simulink model "RecvR4sStEnCtrl1"  (R2024b)
settings: Solver=FixedStepDiscrete  StartTime=0.0  StopTime=10.0  FixedStep=0.01  RelTol=1e-3
model workspace (MAT data in the model file):
  KeSMSw4SSecRwRtStLgrstOtwdInwdClosePos1_Val = Simulink.Parameter
  KeSMSw4SSecRwRtStLgrstOtwdInwdClosePos1_Val.Value = 0
  KeSMSw4SSecRwRtStLgrstOtwdInwdClosePos1_Val.Complexity = 'real'
  KeSMSw4SSecRwRtStLgrstOtwdInwdClosePos1_Val.Dimensions = [1 1]
  KeSMSw4SSecRwRtStLgrstOtwdInwdClosePos1_Val.DataType = 'uint16'
  KeSMSw4SSecRwRtStLgrstUpwdDnwdClosePos1_Val = Simulink.Parameter
  KeSMSw4SSecRwRtStLgrstUpwdDnwdClosePos1_Val.Value = 0
  KeSMSw4SSecRwRtStLgrstUpwdDnwdClosePos1_Val.Complexity = 'real'
  KeSMSw4SSecRwRtStLgrstUpwdDnwdClosePos1_Val.Dimensions = [1 1]
  KeSMSw4SSecRwRtStLgrstUpwdDnwdClosePos1_Val.DataType = 'uint16'
  KeSMSw4SSecRwRtStLgrstUpwdDnwdClosePos2_Val = Simulink.Parameter
  KeSMSw4SSecRwRtStLgrstUpwdDnwdClosePos2_Val.Value = 0
  KeSMSw4SSecRwRtStLgrstUpwdDnwdClosePos2_Val.Complexity = 'real'
  KeSMSw4SSecRwRtStLgrstUpwdDnwdClosePos2_Val.Dimensions = [1 1]
  KeSMSw4SSecRwRtStLgrstUpwdDnwdClosePos2_Val.DataType = 'uint16'
undefined symbols (not defined in the file or in its folder): data, PassStFtEn_Clear, PassStFtEn_Set, SecRwRtStBkReclnEn_Clear, SecRwRtStBkReclnEn_Set, SecRwRtStLgrstUpwdDnwdEn_Clear, SecRwRtStLgrstUpwdDnwdEn_Set
libraries: simulink x1
settings Model: ParameterArgumentNames=KeSMSw4SSecRwRtStLgrstOtwdInwdClosePos1_Val,KeSMSw4SSecRwRtStLgrstUpwdDnwdClosePos1_Val,KeSMSw4SSecRwRtStLgrstUpwdDnwdClosePos2_Val  Creator=sn2xws  LastModifiedBy=sn55gm
settings SolverCC: AlgebraicLoopSolver=TrustRegion
settings DataIOCC: SaveFormat=StructureWithTime  ReturnWorkspaceOutputs=off
settings OptimizationCC: DefaultParameterBehavior=Inlined  EnhancedBackFolding=on  PassReuseOutputArgsAs=Individual arguments  ZeroExternalMemoryAtStartup=off  ZeroInternalMemoryAtStartup=off  OptimizeBlockOrder=speed  DifferentSizesBufferReuse=on  OptimizationCustomize=off  EfficientTunableParamExpr=on
settings DebuggingCC: ParameterTunabilityLossMsg=error  UnconnectedInputMsg=warning  UnconnectedOutputMsg=warning  UnconnectedLineMsg=warning  ArithmeticOperatorsInVariantConditions=warning
settings ModelReferenceCC: EnableRefExpFcnMdlSchedulingChecks=on
settings SFSimCC: MATLABDynamicMemAlloc=off  CustomCodeUndefinedFunction=UseInterfaceOnly
settings RTWCC: Description=AUTOSAR  SystemTargetFile=autosar.tlc  GenCodeOnly=on  TemplateMakefile=ert_default_tmf  GenerateReport=on  IncludeHyperlinkInReport=on  LaunchReport=on  DataTypeReplacement=CDataTypesFixedWidth  GenerateTraceInfo=on  GenerateTraceReport=on  GenerateTraceReportSl=on  GenerateTraceReportSf=on  GenerateTraceReportEml=on  GenerateCodeMetricsReport=on  GPUComputeCapability=3.5
settings CodeAppCC: ForceParamTrailComments=on  IgnoreCustomStorageClasses=off  OperatorAnnotations=on  SimulinkDataObjDesc=on  SFDataObjDesc=on  InsertBlockDesc=on
settings STFCustomTargetCC: TargetLangStandard=C99 (ISO)  MultiwordLength=256  ParMdlRefBuildCompliant=on  CompOptLevelCompliant=on  IncludeMdlTerminateFcn=off  CombineOutputUpdateFcns=on  SuppressErrorStatus=on  ERTCustomFileBanners=on  SupportNonFinite=off  SupportComplex=off  SupportContinuousTime=off  SupportNonInlinedSFcns=off  RemoveResetFunc=on  MATLABClassNameForMDSCustomization=Simulink.SoftwareTarget.ERTCustomization  AutosarCompliant=on  UseToolchainInfoCompliant=on  LookupTableObjectStructAxisOrder=2,1,3,4,...  LUTObjectStructOrderEvenSpacing=Size,Table,Breakpoints  SystemTargetFile=autosar.tlc
settings ERTTargetCC: TargetLangStandard=C99 (ISO)  ConcurrentExecutionCompliant=off  IncludeMdlTerminateFcn=off  SuppressErrorStatus=on  SupportNonFinite=off  SupportComplex=off  ModelStepFunctionPrototypeControlCompliant=off  CPPClassGenCompliant=off  AutosarCompliant=on  LookupTableObjectStructAxisOrder=2,1,3,4,...  LUTObjectStructOrderEvenSpacing=Size,Table,Breakpoints  ERTCustomFileTemplate=example_file_process.tlc  ERTFilePackagingFormat=Compact  BooleanTrueId=TRUE  BooleanFalseId=FALSE  DynamicArrayContainerType=coder::array

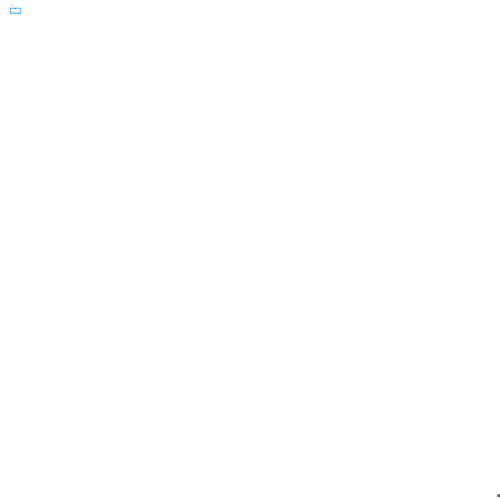
[thumbnail: Simulink's stored preview of the top-level diagram]
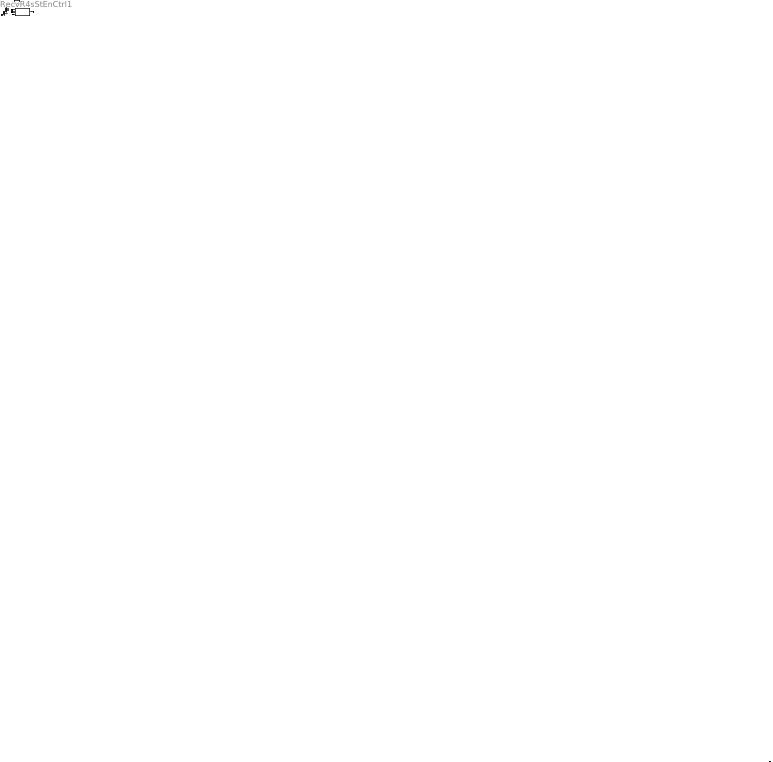
== system RecvR4sStEnCtrl1 ==
  note: Delete block
  note: Delete block
  note: Delete block
  IfVeSMSuRrRtStFtUpwdDnwdPos_Val : Inport  OutDataTypeStr=uint16  PortDimensions=1
  IfVeSMSuSecRwRtStLgrstOtwdInwdPos_Val : Inport  Port=2  OutDataTypeStr=uint16  PortDimensions=1
  IfVeSMSuSecRwRtStLgrstUpwdDnwdPos_Val : Inport  Port=3  OutDataTypeStr=uint16  PortDimensions=1
  MdXXIsTargetPosZone_Val : Inport  Port=4  OutDataTypeStr=uint32  PortDimensions=1
  SecRwRtStBkReclnStgDone_Val : Inport  Port=5  OutDataTypeStr=boolean  PortDimensions=1
  SecRwRtStFtrstStgDone_Val : Inport  Port=6  OutDataTypeStr=boolean  PortDimensions=1
  SecRwRtStHdrstFrwdBkwdStgDone_Val : Inport  Port=7  OutDataTypeStr=boolean  PortDimensions=1
  SecRwRtStHdrstUpwdDnwdStgDone_Val : Inport  Port=8  OutDataTypeStr=boolean  PortDimensions=1
  SecRwRtStLgrstOtwdInwdStgDone_Val : Inport  Port=9  OutDataTypeStr=boolean  PortDimensions=1
  SecRwRtStLgrstUpwdDnwdStgDone_Val : Inport  Port=10  OutDataTypeStr=boolean  PortDimensions=1
  PassSeatOccupied_Val : Inport  Port=11  OutDataTypeStr=boolean  PortDimensions=1
  PassStBkReclnStgDone_Val : Inport  Port=12  OutDataTypeStr=boolean  PortDimensions=1
  PassStFwdBkwdStgDone_Val : Inport  Port=13  OutDataTypeStr=boolean  PortDimensions=1
  RecvR4sStEnCtrl_Init : Subsystem
  RecvRStEnCtrl_Cal_sys : Subsystem
  RecvR4sMdDone_Val : Outport  OutDataTypeStr=uint8  PortDimensions=1  VectorParamsAs1DForOutWhenUnconnected=off
  wires:
  IfVeSMSuRrRtStFtUpwdDnwdPos_Val/1 -> RecvRStEnCtrl_Cal_sys/2(PassStFtStgDone_Val_read)
  IfVeSMSuSecRwRtStLgrstOtwdInwdPos_Val/1 -> ?
  IfVeSMSuSecRwRtStLgrstUpwdDnwdPos_Val/1 -> ?
  MdXXIsTargetPosZone_Val/1 -> RecvRStEnCtrl_Cal_sys/1(MdXXIsTargetPosZone_Val_read)
  SecRwRtStBkReclnStgDone_Val/1 -> RecvRStEnCtrl_Cal_sys/3(SecRwRtStBkReclnStgDone_Val_read)
  SecRwRtStFtrstStgDone_Val/1 -> ?
  SecRwRtStHdrstFrwdBkwdStgDone_Val/1 -> ?
  SecRwRtStHdrstUpwdDnwdStgDone_Val/1 -> ?
  SecRwRtStLgrstOtwdInwdStgDone_Val/1 -> ?
  SecRwRtStLgrstUpwdDnwdStgDone_Val/1 -> RecvRStEnCtrl_Cal_sys/4(SecRwRtStLgrstUpwdDnwdStgDone_Val_read)
  RecvRStEnCtrl_Cal_sys/1(RecvRMdDone_Val_write) -> RecvR4sMdDone_Val/1

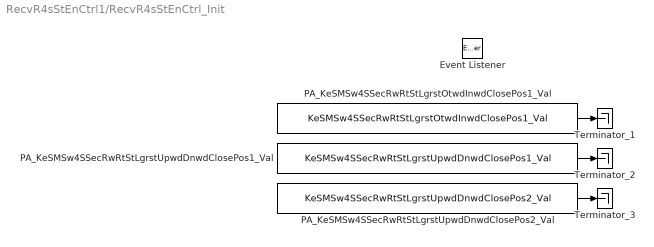
== system RecvR4sStEnCtrl1/RecvR4sStEnCtrl_Init ==
  Event Listener : EventListener  EventName=reset
  PA_KeSMSw4SSecRwRtStLgrstOtwdInwdClosePos1_Val : Constant  Value=KeSMSw4SSecRwRtStLgrstOtwdInwdClosePos1_Val
  PA_KeSMSw4SSecRwRtStLgrstUpwdDnwdClosePos1_Val : Constant  Value=KeSMSw4SSecRwRtStLgrstUpwdDnwdClosePos1_Val
  PA_KeSMSw4SSecRwRtStLgrstUpwdDnwdClosePos2_Val : Constant  Value=KeSMSw4SSecRwRtStLgrstUpwdDnwdClosePos2_Val
  Terminator_1 : Terminator
  Terminator_2 : Terminator
  Terminator_3 : Terminator
  wires:
  PA_KeSMSw4SSecRwRtStLgrstOtwdInwdClosePos1_Val/1 -> Terminator_1/1
  PA_KeSMSw4SSecRwRtStLgrstUpwdDnwdClosePos1_Val/1 -> Terminator_2/1
  PA_KeSMSw4SSecRwRtStLgrstUpwdDnwdClosePos2_Val/1 -> Terminator_3/1

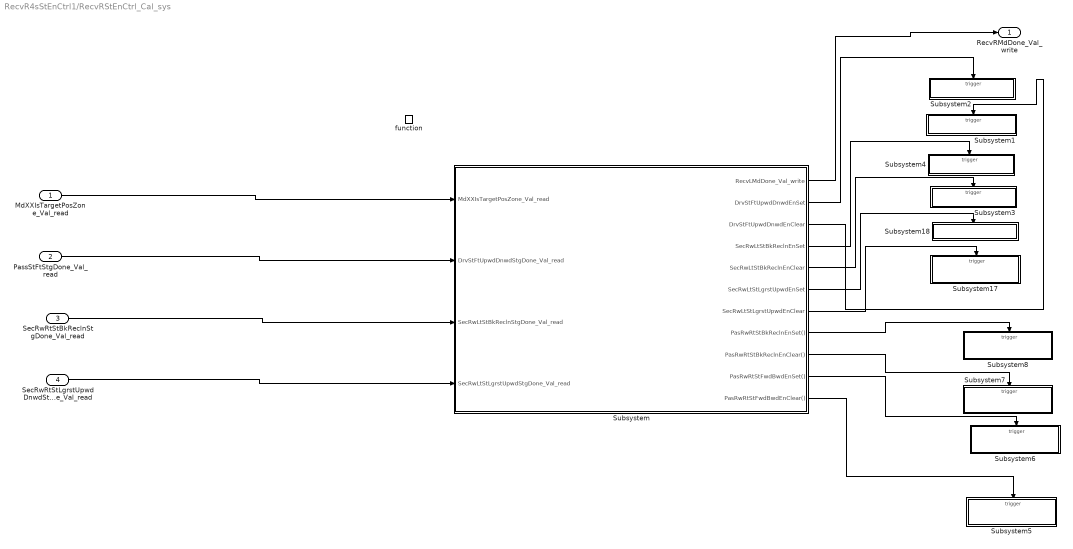
== system RecvR4sStEnCtrl1/RecvRStEnCtrl_Cal_sys ==
  MdXXIsTargetPosZone_Val_read : Inport
  PassStFtStgDone_Val_read : Inport  Port=2
  SecRwRtStBkReclnStgDone_Val_read : Inport  Port=3
  SecRwRtStLgrstUpwdDnwdStgDone_Val_read : Inport  Port=4
  function : TriggerPort  TriggerType=function-call  IsSimulinkFunction=on  FunctionName=RecvR4sStEnCtrl_Cal  VariantControl=(inherit)
  Subsystem : Subsystem
  Subsystem1 : Subsystem
  Subsystem17 : Subsystem
  Subsystem18 : Subsystem
  Subsystem2 : Subsystem
  Subsystem3 : Subsystem
  Subsystem4 : Subsystem
  Subsystem5 : Subsystem
  Subsystem6 : Subsystem
  Subsystem7 : Subsystem
  Subsystem8 : Subsystem
  RecvRMdDone_Val_write : Outport  VectorParamsAs1DForOutWhenUnconnected=off
      settings: EnsureOutportIsVirtual=on
  wires:
  Subsystem/1(RecvLMdDone_Val_write) -> RecvRMdDone_Val_write/1
  MdXXIsTargetPosZone_Val_read/1 -> Subsystem/1(MdXXIsTargetPosZone_Val_read)
  PassStFtStgDone_Val_read/1 -> Subsystem/2(DrvStFtUpwdDnwdStgDone_Val_read)
  SecRwRtStBkReclnStgDone_Val_read/1 -> Subsystem/3(SecRwLtStBkReclnStgDone_Val_read)
  SecRwRtStLgrstUpwdDnwdStgDone_Val_read/1 -> Subsystem/4(SecRwLtStLgrstUpwdStgDone_Val_read)
  Subsystem/7(SecRwLtStLgrstUpwdEnClear) -> Subsystem17/Trigger
  Subsystem/6(SecRwLtStLgrstUpwdEnSet) -> Subsystem18/Trigger
  Subsystem/2(DrvStFtUpwdDnwdEnSet) -> Subsystem2/Trigger
  Subsystem/5(SecRwLtStBkReclnEnClear) -> Subsystem3/Trigger
  Subsystem/3(DrvStFtUpwdDnwdEnClear) -> Subsystem1/Trigger
  Subsystem/4(SecRwLtStBkReclnEnSet) -> Subsystem4/Trigger
  Subsystem/8(PasRwRtStBkReclnEnSet()) -> Subsystem8/Trigger
  Subsystem/9(PasRwRtStBkReclnEnClear()) -> Subsystem7/Trigger
  Subsystem/10(PasRwRtStFwdBwdEnSet()) -> Subsystem6/Trigger
  Subsystem/11(PasRwRtStFwdBwdEnClear()) -> Subsystem5/Trigger

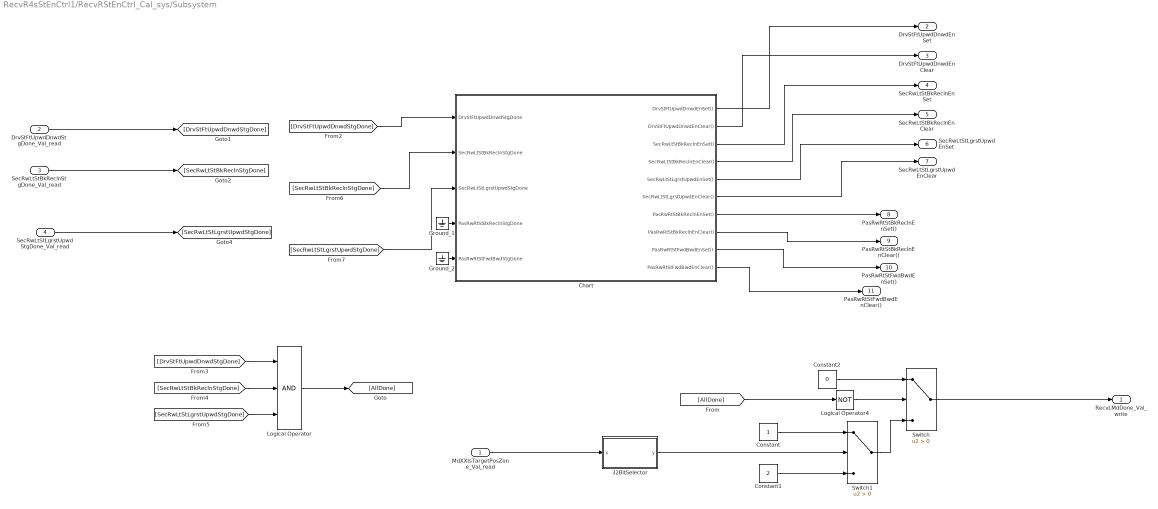
== system RecvR4sStEnCtrl1/RecvRStEnCtrl_Cal_sys/Subsystem ==
  MdXXIsTargetPosZone_Val_read : Inport
  DrvStFtUpwdDnwdStgDone_Val_read : Inport  Port=2
  SecRwLtStBkReclnStgDone_Val_read : Inport  Port=3
  SecRwLtStLgrstUpwdStgDone_Val_read : Inport  Port=4
  32BitSelector : Subsystem  mask(32 Bit Selector){BitNum=12}
      mask prompts: BitNum "Select Bit Number"
      mask help: Allows selection of a particular bit (0-31) out of a packed word up to 32 bits long. Output will be true if the bit number selected via the mask parameter is equal to one.
      mask TypeOptions BitNum: 0 | 1 | 2 | 3 | 4 | 5 | 6 | 7 | 8 | 9 | 10 | 11 | 12 | 13 | 14 | 15 | 16 | 17 | 18 | 19 | 20 | 21 | 22 | 23 | 24 | 25 | 26 | 27 | 28 | 29 | 30 | 31
      mask Display:
      | text(0.5, 0.8,'BIT','horizontalAlignment','center')
      | text(0.5, 0.5,'SELECTOR','horizontalAlignment','center')
      | text(0.5, 0.2,['-- Bit ',char(get_param(gcb,'BitNum')),' --'],'horizontalAlignment','center')
  Chart : Stateflow chart  TreatAsAtomicUnit=on
  Constant : Constant  OutDataTypeStr=uint8
  Constant1 : Constant  Value=2  OutDataTypeStr=uint8
  Constant2 : Constant  Value=0  OutDataTypeStr=uint8
  Ground_1 : Ground
  Ground_2 : Ground
  Logical Operator : Logic  Inputs=3  AllPortsSameDT=off  OutDataTypeStr=boolean
  Logical Operator4 : Logic  Operator=NOT  AllPortsSameDT=off  OutDataTypeStr=boolean
  Switch : Switch  Criteria=u2 > Threshold  SaturateOnIntegerOverflow=off  InputSameDT=off
  Switch1 : Switch  Criteria=u2 > Threshold  SaturateOnIntegerOverflow=off  InputSameDT=off
  RecvLMdDone_Val_write : Outport  VectorParamsAs1DForOutWhenUnconnected=off
      settings: EnsureOutportIsVirtual=on
  DrvStFtUpwdDnwdEnSet : Outport  Port=2  VectorParamsAs1DForOutWhenUnconnected=off
  DrvStFtUpwdDnwdEnClear : Outport  Port=3  VectorParamsAs1DForOutWhenUnconnected=off
  SecRwLtStBkReclnEnSet : Outport  Port=4  VectorParamsAs1DForOutWhenUnconnected=off
  SecRwLtStBkReclnEnClear : Outport  Port=5  VectorParamsAs1DForOutWhenUnconnected=off
  SecRwLtStLgrstUpwdEnSet : Outport  Port=6  VectorParamsAs1DForOutWhenUnconnected=off
  SecRwLtStLgrstUpwdEnClear : Outport  Port=7  VectorParamsAs1DForOutWhenUnconnected=off
  PasRwRtStBkReclnEnSet() : Outport  Port=8
  PasRwRtStBkReclnEnClear() : Outport  Port=9
  PasRwRtStFwdBwdEnSet() : Outport  Port=10
  PasRwRtStFwdBwdEnClear() : Outport  Port=11
  wires:
  Switch/1 -> RecvLMdDone_Val_write/1
  MdXXIsTargetPosZone_Val_read/1 -> 32BitSelector/1(x)
  Switch1/1 -> Switch/3
  DrvStFtUpwdDnwdStgDone_Val_read/1 -> [DrvStFtUpwdDnwdStgDone]
  SecRwLtStBkReclnStgDone_Val_read/1 -> [SecRwLtStBkReclnStgDone]
  SecRwLtStLgrstUpwdStgDone_Val_read/1 -> [SecRwLtStLgrstUpwdStgDone]
  [DrvStFtUpwdDnwdStgDone] -> Logical Operator/1
  [SecRwLtStBkReclnStgDone] -> Logical Operator/2
  [SecRwLtStLgrstUpwdStgDone] -> Logical Operator/3
  Logical Operator/1 -> [AllDone]
  [DrvStFtUpwdDnwdStgDone] -> Chart/1(DrvStFtUpwdDnwdStgDone)
  [SecRwLtStBkReclnStgDone] -> Chart/2(SecRwLtStBkReclnStgDone)
  [SecRwLtStLgrstUpwdStgDone] -> Chart/3(SecRwLtStLgrstUpwdStgDone)
  Chart/1(DrvStFtUpwdDnwdEnSet()) -> DrvStFtUpwdDnwdEnSet/1
  Chart/2(DrvStFtUpwdDnwdEnClear()) -> DrvStFtUpwdDnwdEnClear/1
  Chart/3(SecRwLtStBkReclnEnSet()) -> SecRwLtStBkReclnEnSet/1
  Chart/4(SecRwLtStBkReclnEnClear()) -> SecRwLtStBkReclnEnClear/1
  Chart/5(SecRwLtStLgrstUpwdEnSet()) -> SecRwLtStLgrstUpwdEnSet/1
  Chart/6(SecRwLtStLgrstUpwdEnClear()) -> SecRwLtStLgrstUpwdEnClear/1
  Constant2/1 -> Switch/1
  Constant1/1 -> Switch1/3
  Constant/1 -> Switch1/1
  [AllDone] -> Logical Operator4/1
  Logical Operator4/1 -> Switch/2
  32BitSelector/1(y) -> Switch1/2
  Chart/7(PasRwRtStBkReclnEnSet()) -> PasRwRtStBkReclnEnSet()/1
  Chart/8(PasRwRtStBkReclnEnClear()) -> PasRwRtStBkReclnEnClear()/1
  Chart/9(PasRwRtStFwdBwdEnSet()) -> PasRwRtStFwdBwdEnSet()/1
  Chart/10(PasRwRtStFwdBwdEnClear()) -> PasRwRtStFwdBwdEnClear()/1
  Ground_1/1 -> Chart/4(PasRwRtStBkReclnStgDone)
  Ground_2/1 -> Chart/5(PasRwRtStFwdBwdStgDone)

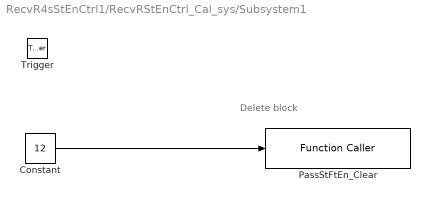
== system RecvR4sStEnCtrl1/RecvRStEnCtrl_Cal_sys/Subsystem1 ==
  note: Delete block
  Trigger : TriggerPort  TriggerType=function-call  VariantControl=Variant  PortDimensions=1
  Constant : Constant  Value=12  OutDataTypeStr=uint8
  PassStFtEn_Clear : FunctionCaller  FunctionPrototype=PassStFtEn_Clear(data)  InputArgumentSpecifications=uint8(1)  OutputArgumentSpecifications=<Enter example>
  wires:
  Constant/1 -> PassStFtEn_Clear/1

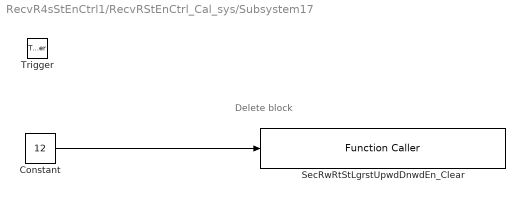
== system RecvR4sStEnCtrl1/RecvRStEnCtrl_Cal_sys/Subsystem17 ==
  note: Delete block
  Trigger : TriggerPort  TriggerType=function-call  VariantControl=Variant  PortDimensions=1
  Constant : Constant  Value=12  OutDataTypeStr=uint8
  SecRwRtStLgrstUpwdDnwdEn_Clear : FunctionCaller  FunctionPrototype=SecRwRtStLgrstUpwdDnwdEn_Clear(data)  InputArgumentSpecifications=uint8(1)  OutputArgumentSpecifications=<Enter example>
  wires:
  Constant/1 -> SecRwRtStLgrstUpwdDnwdEn_Clear/1

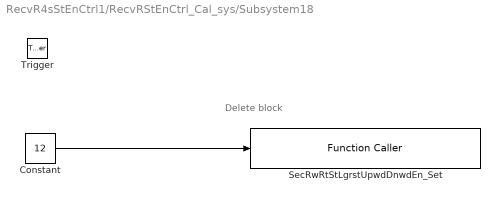
== system RecvR4sStEnCtrl1/RecvRStEnCtrl_Cal_sys/Subsystem18 ==
  note: Delete block
  Trigger : TriggerPort  TriggerType=function-call  VariantControl=Variant  PortDimensions=1
  Constant : Constant  Value=12  OutDataTypeStr=uint8
  SecRwRtStLgrstUpwdDnwdEn_Set : FunctionCaller  FunctionPrototype=SecRwRtStLgrstUpwdDnwdEn_Set(data)  InputArgumentSpecifications=uint8(1)  OutputArgumentSpecifications=<Enter example>
  wires:
  Constant/1 -> SecRwRtStLgrstUpwdDnwdEn_Set/1

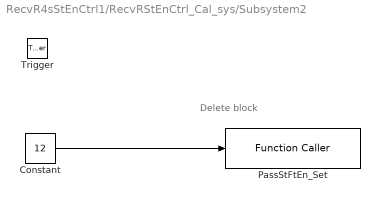
== system RecvR4sStEnCtrl1/RecvRStEnCtrl_Cal_sys/Subsystem2 ==
  note: Delete block
  Trigger : TriggerPort  TriggerType=function-call  VariantControl=Variant  PortDimensions=1
  Constant : Constant  Value=12  OutDataTypeStr=uint8
  PassStFtEn_Set : FunctionCaller  FunctionPrototype=PassStFtEn_Set(data)  InputArgumentSpecifications=uint8(1)  OutputArgumentSpecifications=<Enter example>
  wires:
  Constant/1 -> PassStFtEn_Set/1

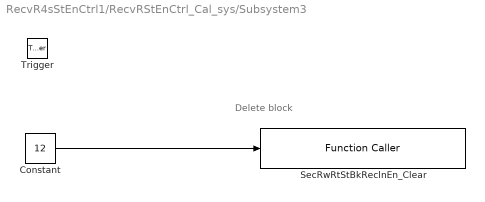
== system RecvR4sStEnCtrl1/RecvRStEnCtrl_Cal_sys/Subsystem3 ==
  note: Delete block
  Trigger : TriggerPort  TriggerType=function-call  VariantControl=Variant  PortDimensions=1
  Constant : Constant  Value=12  OutDataTypeStr=uint8
  SecRwRtStBkReclnEn_Clear : FunctionCaller  FunctionPrototype=SecRwRtStBkReclnEn_Clear(data)  InputArgumentSpecifications=uint8(1)  OutputArgumentSpecifications=<Enter example>
  wires:
  Constant/1 -> SecRwRtStBkReclnEn_Clear/1

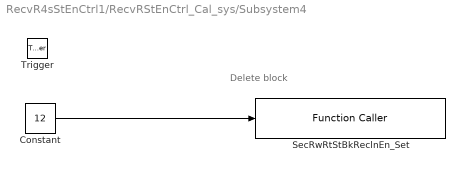
== system RecvR4sStEnCtrl1/RecvRStEnCtrl_Cal_sys/Subsystem4 ==
  note: Delete block
  Trigger : TriggerPort  TriggerType=function-call  VariantControl=Variant  PortDimensions=1
  Constant : Constant  Value=12  OutDataTypeStr=uint8
  SecRwRtStBkReclnEn_Set : FunctionCaller  FunctionPrototype=SecRwRtStBkReclnEn_Set(data)  InputArgumentSpecifications=uint8(1)  OutputArgumentSpecifications=<Enter example>
  wires:
  Constant/1 -> SecRwRtStBkReclnEn_Set/1

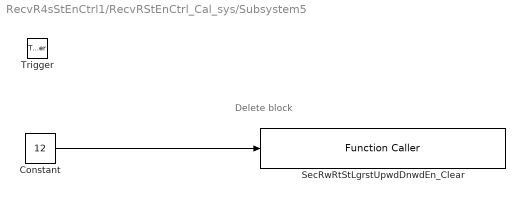
== system RecvR4sStEnCtrl1/RecvRStEnCtrl_Cal_sys/Subsystem5 ==
  note: Delete block
  Trigger : TriggerPort  TriggerType=function-call  VariantControl=Variant  PortDimensions=1
  Constant : Constant  Value=12  OutDataTypeStr=uint8
  SecRwRtStLgrstUpwdDnwdEn_Clear : FunctionCaller  FunctionPrototype=SecRwRtStLgrstUpwdDnwdEn_Clear(data)  InputArgumentSpecifications=uint8(1)  OutputArgumentSpecifications=<Enter example>
  wires:
  Constant/1 -> SecRwRtStLgrstUpwdDnwdEn_Clear/1

== system RecvR4sStEnCtrl1/RecvRStEnCtrl_Cal_sys/Subsystem6 ==
  note: Delete block
  Trigger : TriggerPort  TriggerType=function-call  VariantControl=Variant  PortDimensions=1
  Constant : Constant  Value=12  OutDataTypeStr=uint8
  SecRwRtStLgrstUpwdDnwdEn_Clear : FunctionCaller  FunctionPrototype=SecRwRtStLgrstUpwdDnwdEn_Clear(data)  InputArgumentSpecifications=uint8(1)  OutputArgumentSpecifications=<Enter example>
  wires:
  Constant/1 -> SecRwRtStLgrstUpwdDnwdEn_Clear/1

== system RecvR4sStEnCtrl1/RecvRStEnCtrl_Cal_sys/Subsystem7 ==
  note: Delete block
  Trigger : TriggerPort  TriggerType=function-call  VariantControl=Variant  PortDimensions=1
  Constant : Constant  Value=12  OutDataTypeStr=uint8
  SecRwRtStLgrstUpwdDnwdEn_Clear : FunctionCaller  FunctionPrototype=SecRwRtStLgrstUpwdDnwdEn_Clear(data)  InputArgumentSpecifications=uint8(1)  OutputArgumentSpecifications=<Enter example>
  wires:
  Constant/1 -> SecRwRtStLgrstUpwdDnwdEn_Clear/1

== system RecvR4sStEnCtrl1/RecvRStEnCtrl_Cal_sys/Subsystem8 ==
  note: Delete block
  Trigger : TriggerPort  TriggerType=function-call  VariantControl=Variant  PortDimensions=1
  Constant : Constant  Value=12  OutDataTypeStr=uint8
  SecRwRtStLgrstUpwdDnwdEn_Clear : FunctionCaller  FunctionPrototype=SecRwRtStLgrstUpwdDnwdEn_Clear(data)  InputArgumentSpecifications=uint8(1)  OutputArgumentSpecifications=<Enter example>
  wires:
  Constant/1 -> SecRwRtStLgrstUpwdDnwdEn_Clear/1

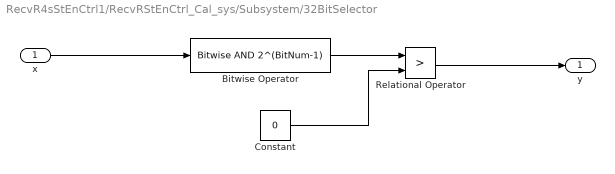
== system RecvR4sStEnCtrl1/RecvRStEnCtrl_Cal_sys/Subsystem/32BitSelector ==
  x : Inport
  Bitwise Operator : simulink/Logic and Bit Operations/Bitwise Operator  logicop=AND  UseBitMask=on  BitMask=2^(BitNum-1)  BitMaskRealWorld=Stored Integer
  Constant : Constant  Value=0  OutDataTypeStr=uint32
  Relational Operator : RelationalOperator  Operator=>  OutDataTypeStr=boolean  RndMeth=Simplest  InputSameDT=off
  y : Outport  VectorParamsAs1DForOutWhenUnconnected=off
  wires:
  Relational Operator/1 -> y/1
  Constant/1 -> Relational Operator/2
  x/1 -> Bitwise Operator/1
  Bitwise Operator/1 -> Relational Operator/1

== stateflow chart RecvR4sStEnCtrl1/RecvRStEnCtrl_Cal_sys/Subsystem/Chart ==
  (default) -> (junction 11)
  (junction 11) -> (junction 13)
  (junction 13) -> (junction 15) [order 1] : [DrvStFtUpwdDnwdStgDone]
  (junction 13) -> (junction 19) [order 2] : {DrvStFtUpwdDnwdEnSet;}
  (junction 15) -> (junction 17) : {DrvStFtUpwdDnwdEnClear;}
  (junction 17) -> (junction 19)
  (junction 19) -> (junction 24)
  (junction 24) -> (junction 26) [order 1] : [SecRwLtStBkReclnStgDone]
  (junction 24) -> (junction 30) [order 2] : {SecRwLtStBkReclnEnSet;}
  (junction 26) -> (junction 28) : {SecRwLtStBkReclnEnClear;}
  (junction 28) -> (junction 30)
  (junction 30) -> (junction 34)
  (junction 34) -> (junction 36) [order 1] : [SecRwLtStLgrstUpwdStgDone]
  (junction 36) -> (junction 43) : {SecRwLtStLgrstUpwdEnClear;}
  (junction 34) -> (junction 40) [order 2] : {SecRwLtStLgrstUpwdEnSet;}
  (junction 43) -> (junction 44) [order 1] : [PasRwRtStBkReclnStgDone]
  (junction 43) -> (junction 46) [order 2] : {PasRwRtStBkReclnEnSet;}
  (junction 44) -> (junction 45) : {PasRwRtStBkReclnEnClear;}
  (junction 45) -> (junction 46)
  (junction 46) -> (junction 53)
  (junction 53) -> (junction 55) [order 1] : [PasRwRtStFwdBwdStgDone]
  (junction 55) -> (junction 47) : {PasRwRtStFwdBwdEnClear;}
  (junction 53) -> (junction 38) [order 2] : {PasRwRtStFwdBwdEnSet;}
  (junction 47) -> (junction 38)
  (junction 38) -> (junction 40)
  data: DrvStFtUpwdDnwdStgDone input; SecRwLtStBkReclnStgDone input; SecRwLtStLgrstUpwdStgDone input; PasRwRtStBkReclnStgDone input; PasRwRtStFwdBwdStgDone input
  events: DrvStFtUpwdDnwdEnSet output FUNCTION_CALL_EVENT; DrvStFtUpwdDnwdEnClear output FUNCTION_CALL_EVENT; SecRwLtStBkReclnEnSet output FUNCTION_CALL_EVENT; SecRwLtStBkReclnEnClear output FUNCTION_CALL_EVENT; SecRwLtStLgrstUpwdEnSet output FUNCTION_CALL_EVENT; SecRwLtStLgrstUpwdEnClear output FUNCTION_CALL_EVENT; PasRwRtStBkReclnEnSet output FUNCTION_CALL_EVENT; PasRwRtStBkReclnEnClear output FUNCTION_CALL_EVENT; PasRwRtStFwdBwdEnSet output FUNCTION_CALL_EVENT; PasRwRtStFwdBwdEnClear output FUNCTION_CALL_EVENT
